simulink model "PID"  (R2018a)
settings: Solver=VariableStepAuto  StartTime=0.0  StopTime=30  RelTol=1e-3
libraries: simulink x6
settings Model: Creator=rahul  LastModifiedBy=rahul

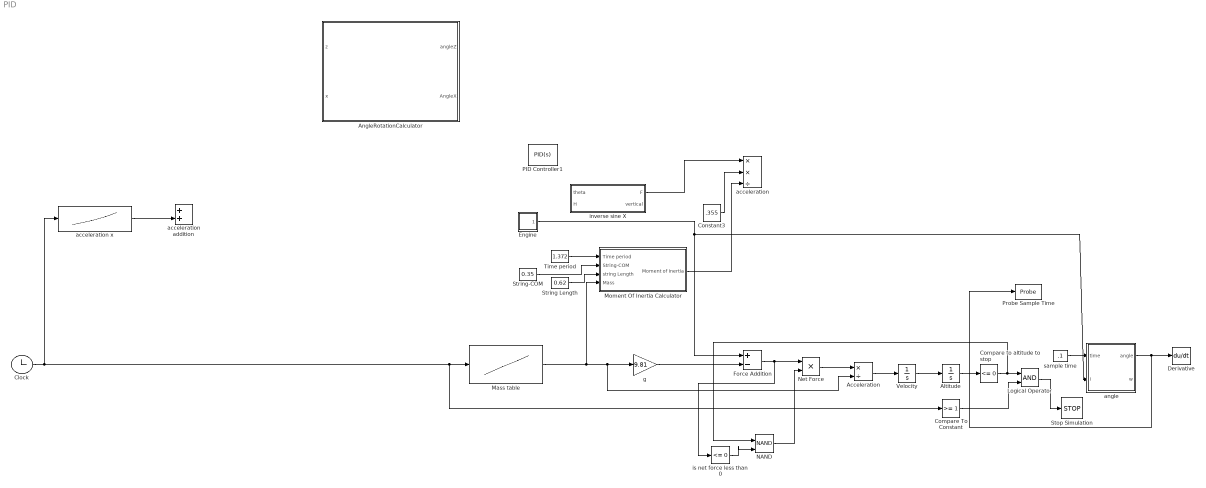
== system PID ==
  Acceleration : Product  Inputs=*/
  Altitude : Integrator  LimitOutput=on  LowerSaturationLimit=0
  AngleRotationCalculator : Subsystem
  Clock : Clock
  Compare To Constant : simulink/Logic and Bit Operations/Compare To Constant  relop=>=  const=1  OutDataTypeStr=boolean
  Compare to altitude to stop : simulink/Logic and Bit Operations/Compare To Constant  relop=<=  const=0  OutDataTypeStr=boolean
  Constant3 : Constant  Value=.355
  Derivative : Derivative
  Engine : Subsystem
  Force Addition : Sum  Inputs=+-
  Logical Operator : Logic  AllPortsSameDT=off  OutDataTypeStr=boolean
  Mass table : Lookup  InputValues=[0,1]  Table=[0.975,.8]  LookUpMeth=Use Input Nearest  SaturateOnIntegerOverflow=on
  Moment Of Inertia Calculator : Subsystem
  NAND : Logic  Operator=NAND  IconShape=distinctive  AllPortsSameDT=off  OutDataTypeStr=boolean
  Net Force : Product  Inputs=**
  PID Controller1 : simulink/Continuous/PID Controller  Controller=PID  TimeDomain=Continuous-time  SampleTime=-1  IntegratorMethod=Forward Euler  FilterMethod=Forward Euler  Form=Parallel  UseFilter=on  ControllerParametersSource=internal  P=0  I=0.000379361726906509  D=0  N=100  InitialConditionSource=internal  InitialConditionForIntegrator=0  InitialConditionForFilter=0  ExternalReset=none  LimitOutput=on  UpperSaturationLimit=0.0872664626  LowerSaturationLimit=-0.0872664626  LinearizeAsGain=on  AntiWindupMode=none  Kb=1  TrackingMode=off  Kt=1  PParamMin=[]  PParamMax=[]  IParamMin=[]  IParamMax=[]  DParamMin=[]  DParamMax=[]  NParamMin=[]  NParamMax=[]  KbParamMin=[]  KbParamMax=[]  KtParamMin=[]  KtParamMax=[]  POutMin=[]  POutMax=[]  IOutMin=[]  IOutMax=[]  DOutMin=[]  DOutMax=[]  NOutMin=[]  NOutMax=[]  KbOutMin=[]  KbOutMax=[]  KtOutMin=[]  KtOutMax=[]  IntegratorOutMin=[]  IntegratorOutMax=[]  FilterOutMin=[]  FilterOutMax=[]  SumOutMin=[]  SumOutMax=[]  SumI1OutMin=[]  SumI1OutMax=[]  SumI2OutMin=[]  SumI2OutMax=[]  SumI3OutMin=[]  SumI3OutMax=[]  SumDOutMin=[]  SumDOutMax=[]  SaturationOutMin=[]  SaturationOutMax=[]  IntegratorContinuousStateAttributes=''  IntegratorStateMustResolveToSignalObject=off  IntegratorRTWStateStorageClass=Auto  FilterContinuousStateAttributes=''  FilterStateMustResolveToSignalObject=off  FilterRTWStateStorageClass=Auto  DifferentiatorICPrevScaledInput=0  DifferentiatorOutMin=[]  DifferentiatorOutMax=[]  FilterDiffOutCoefMin=[]  FilterDiffOutCoefMax=[]  SumDenOutMin=[]  SumDenOutMax=[]  SumNumOutMin=[]  SumNumOutMax=[]  ReciprocalOutMin=[]  ReciprocalOutMax=[]  DivideOutMin=[]  DivideOutMax=[]  TunerSelectOption=Transfer Function Based (PID Tuner App)
  Probe Sample Time : Probe  ProbeWidth=off  ProbeComplexSignal=off
  Stop Simulation : Stop
  String Length : Constant  Value=0.62
  String-COM : Constant  Value=0.35
  Time period : Constant  Value=1.372
  Velocity : Integrator
  acceleration : Product  Inputs=**/
  acceleration addition : Sum
  acceleration x : Lookup  InputValues=[0,1.5,3]  Table=[0, 0.2,0]  LookUpMeth=Interpolation-Use End Values  SaturateOnIntegerOverflow=on
  angle : MATLAB Function  TreatAsAtomicUnit=on
  g : Gain  Gain=9.81
  inverse sine X : MATLAB Function  TreatAsAtomicUnit=on  SystemSampleTime=.001
  is net force less than 0 : simulink/Logic and Bit Operations/Compare To Constant  relop=<=  const=0  OutDataTypeStr=boolean
  sample time : Constant  Value=.1
  wires:
  Force Addition/1 -> is net force less than 0/1, Net Force/1
  NAND/1 -> Net Force/2
  Logical Operator/1 -> Stop Simulation/1
  g/1 -> Force Addition/2
  Time period/1 -> Moment Of Inertia Calculator/1(Time period)
  String-COM/1 -> Moment Of Inertia Calculator/2(String-COM)
  Net Force/1 -> Acceleration/1
  Clock/1 -> Compare To Constant/1, Mass table/1, acceleration x/1
  Compare To Constant/1 -> Logical Operator/2
  Acceleration/1 -> Velocity/1
  Compare to altitude to stop/1 -> NAND/1, Logical Operator/1
  Velocity/1 -> Altitude/1
  String Length/1 -> Moment Of Inertia Calculator/3(string Length)
  Mass table/1 -> Moment Of Inertia Calculator/4(Mass), Acceleration/2, g/1
  Altitude/1 -> Compare to altitude to stop/1
  Constant3/1 -> acceleration/2
  inverse sine X/1(F) -> acceleration/1
  Moment Of Inertia Calculator/1(Moment of Inertia) -> acceleration/3
  acceleration x/1 -> acceleration addition/2
  sample time/1 -> angle/1(time)
  angle/1(angle) -> Probe Sample Time/1, Derivative/1
  Engine/1(Thrust) -> angle/2(i), Force Addition/1
  is net force less than 0/1 -> NAND/2

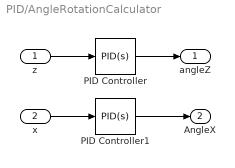
== system PID/AngleRotationCalculator ==
  z : Inport
  x : Inport  Port=2
  PID Controller : simulink/Continuous/PID Controller  Controller=PID  TimeDomain=Continuous-time  SampleTime=-1  IntegratorMethod=Forward Euler  FilterMethod=Forward Euler  Form=Parallel  UseFilter=on  ControllerParametersSource=internal  P=1  I=1  D=0  N=100  InitialConditionSource=internal  InitialConditionForIntegrator=0  InitialConditionForFilter=0  ExternalReset=none  LimitOutput=off  UpperSaturationLimit=inf  LowerSaturationLimit=-inf  LinearizeAsGain=on  AntiWindupMode=none  Kb=1  TrackingMode=off  Kt=1  PParamMin=[]  PParamMax=[]  IParamMin=[]  IParamMax=[]  DParamMin=[]  DParamMax=[]  NParamMin=[]  NParamMax=[]  KbParamMin=[]  KbParamMax=[]  KtParamMin=[]  KtParamMax=[]  POutMin=[]  POutMax=[]  IOutMin=[]  IOutMax=[]  DOutMin=[]  DOutMax=[]  NOutMin=[]  NOutMax=[]  KbOutMin=[]  KbOutMax=[]  KtOutMin=[]  KtOutMax=[]  IntegratorOutMin=[]  IntegratorOutMax=[]  FilterOutMin=[]  FilterOutMax=[]  SumOutMin=[]  SumOutMax=[]  SumI1OutMin=[]  SumI1OutMax=[]  SumI2OutMin=[]  SumI2OutMax=[]  SumI3OutMin=[]  SumI3OutMax=[]  SumDOutMin=[]  SumDOutMax=[]  SaturationOutMin=[]  SaturationOutMax=[]  IntegratorContinuousStateAttributes=''  IntegratorStateMustResolveToSignalObject=off  IntegratorRTWStateStorageClass=Auto  FilterContinuousStateAttributes=''  FilterStateMustResolveToSignalObject=off  FilterRTWStateStorageClass=Auto  DifferentiatorICPrevScaledInput=0  DifferentiatorOutMin=[]  DifferentiatorOutMax=[]  FilterDiffOutCoefMin=[]  FilterDiffOutCoefMax=[]  SumDenOutMin=[]  SumDenOutMax=[]  SumNumOutMin=[]  SumNumOutMax=[]  ReciprocalOutMin=[]  ReciprocalOutMax=[]  DivideOutMin=[]  DivideOutMax=[]  TunerSelectOption=Transfer Function Based (PID Tuner App)
  PID Controller1 : simulink/Continuous/PID Controller  Controller=PID  TimeDomain=Continuous-time  SampleTime=-1  IntegratorMethod=Forward Euler  FilterMethod=Forward Euler  Form=Parallel  UseFilter=on  ControllerParametersSource=internal  P=0  I=-1  D=0  N=100  InitialConditionSource=internal  InitialConditionForIntegrator=0  InitialConditionForFilter=0  ExternalReset=none  LimitOutput=on  UpperSaturationLimit=-0.0872664626  LowerSaturationLimit=-0.0872664626  LinearizeAsGain=on  AntiWindupMode=none  Kb=1  TrackingMode=off  Kt=1  PParamMin=[]  PParamMax=[]  IParamMin=[]  IParamMax=[]  DParamMin=[]  DParamMax=[]  NParamMin=[]  NParamMax=[]  KbParamMin=[]  KbParamMax=[]  KtParamMin=[]  KtParamMax=[]  POutMin=[]  POutMax=[]  IOutMin=[]  IOutMax=[]  DOutMin=[]  DOutMax=[]  NOutMin=[]  NOutMax=[]  KbOutMin=[]  KbOutMax=[]  KtOutMin=[]  KtOutMax=[]  IntegratorOutMin=[]  IntegratorOutMax=[]  FilterOutMin=[]  FilterOutMax=[]  SumOutMin=[]  SumOutMax=[]  SumI1OutMin=[]  SumI1OutMax=[]  SumI2OutMin=[]  SumI2OutMax=[]  SumI3OutMin=[]  SumI3OutMax=[]  SumDOutMin=[]  SumDOutMax=[]  SaturationOutMin=[]  SaturationOutMax=[]  IntegratorContinuousStateAttributes=''  IntegratorStateMustResolveToSignalObject=off  IntegratorRTWStateStorageClass=Auto  FilterContinuousStateAttributes=''  FilterStateMustResolveToSignalObject=off  FilterRTWStateStorageClass=Auto  DifferentiatorICPrevScaledInput=0  DifferentiatorOutMin=[]  DifferentiatorOutMax=[]  FilterDiffOutCoefMin=[]  FilterDiffOutCoefMax=[]  SumDenOutMin=[]  SumDenOutMax=[]  SumNumOutMin=[]  SumNumOutMax=[]  ReciprocalOutMin=[]  ReciprocalOutMax=[]  DivideOutMin=[]  DivideOutMax=[]  TunerSelectOption=Transfer Function Based (PID Tuner App)
  angleZ : Outport
  AngleX : Outport  Port=2
  wires:
  PID Controller1/1 -> AngleX/1
  PID Controller/1 -> angleZ/1
  x/1 -> PID Controller1/1
  z/1 -> PID Controller/1

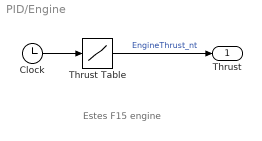
== system PID/Engine ==
  note: Estes F15 engine
  Clock : Clock
  Thrust Table : Lookup  InputValues=|  Table=[0,12.5,25,16.5,15.25,15,14.5,14.5,14.25,14,13,13,0]  LookUpMeth=Interpolation-Use End Values  SaturateOnIntegerOverflow=on
      | [0,
      | 0.25,
      | 0.5,
      | 0.75,
      | 1,
      | 1.25,
      | 1.5,
      | 2,
      | 2.25,
      | 2.5,
      | 3,
      | 3.25,
      | 3.5]
  Thrust : Outport
  wires:
  Clock/1 -> Thrust Table/1
  Thrust Table/1 -> Thrust/1  "EngineThrust_nt"

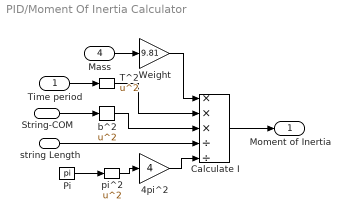
== system PID/Moment Of Inertia Calculator ==
  Time period : Inport
  String-COM : Inport  Port=2
  string Length : Inport  Port=3
  Mass : Inport  Port=4
  4pi^2 : Gain  Gain=4
  Calculate I : Product  Inputs=***//
  Pi : Constant  Value=pi
  T^2 : Math  Operator=square  SaturateOnIntegerOverflow=on
  Weight : Gain  Gain=9.81
  b^2 : Math  Operator=square  SaturateOnIntegerOverflow=on
  pi^2 : Math  Operator=square  SaturateOnIntegerOverflow=on
  Moment of Inertia : Outport
  wires:
  Time period/1 -> T^2/1
  Calculate I/1 -> Moment of Inertia/1
  string Length/1 -> Calculate I/4
  Mass/1 -> Weight/1
  Weight/1 -> Calculate I/1
  pi^2/1 -> 4pi^2/1
  b^2/1 -> Calculate I/3
  T^2/1 -> Calculate I/2
  String-COM/1 -> b^2/1
  Pi/1 -> pi^2/1
  4pi^2/1 -> Calculate I/5

== matlab function PID/angle ==
  settings: updateMethod=DISCRETE
  data: angle output; time input; w output; i input
function [angle, w]= inverseSine(time, i)
    af = 0;
    ai = 0;
    wi = 0;
    
    while 1
        %{
        if i == 0
            break
        end
        wi = (2 * (af - ai) / time) - wi;
        w = wi;

        ai = af;
        af = 2 * ai + 5;
        %}
        angle = 5;
    end 
    
    angle = af;
    w = 0;

== matlab function PID/inverse sine X ==
  data: theta input; F output; H input; vertical output
function [F, vertical]  = inverseSine(theta, H)
    F = H * sin(theta);
    vertical = H * cos(theta);
